simulink model "estimation"  (R2024a)
settings: Solver=VariableStepAuto  StartTime=0.0  StopTime=800  RelTol=1e-3
settings Model: NumberOfSteps=2  Creator=sabri  LastModifiedBy=sabri

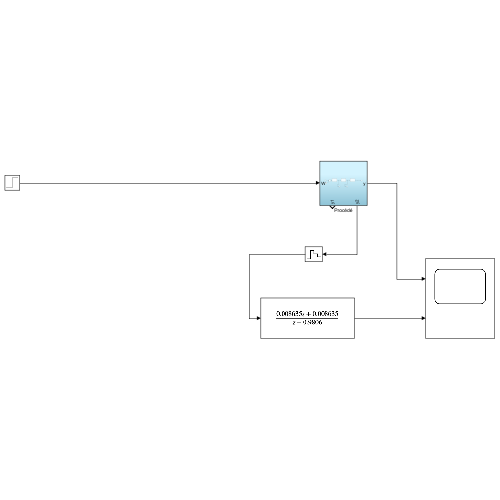
[thumbnail: Simulink's stored preview of the top-level diagram]
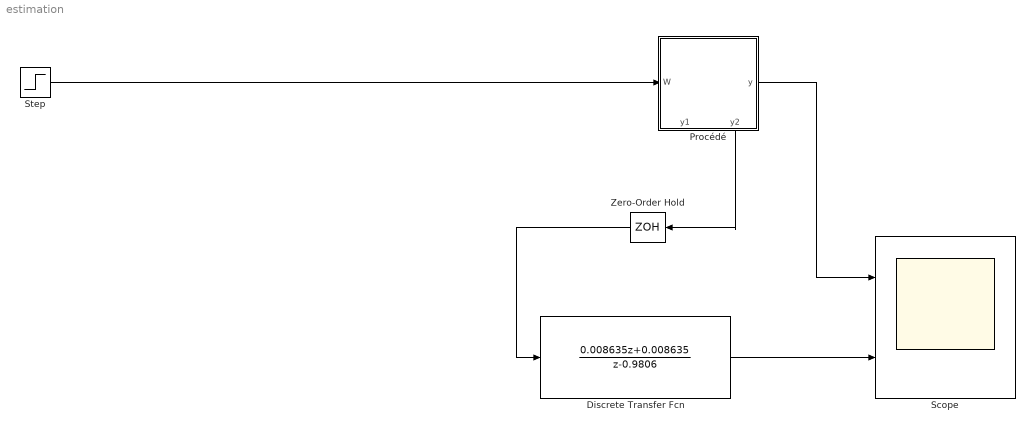
== system estimation ==
  Discrete Transfer Fcn : DiscreteTransferFcn  Numerator=[0.008635 0.008635]  Denominator=[1 -0.9806]
  Procédé : Subsystem
      settings: PortSchema="{\"entries\":[{\"content\":{\"sides\":[{\"content\":{\"connectorIds\":[\"In1\"]},\"type\":\"ConnectorPlacement.EquallySpacedRectSide\",\"uuid\":\"20a23230-a41b-4fdf-8ae4-039aa17abee7\"},{\"content\":{\"connectorIds\":[\"Out1\"],\"side\":\"RIGHT\"},\"type\":\"ConnectorPlacement.EquallySpacedRectSide\",\"uuid\":\"82e4e468-e0ad-4c9f-b6ff-cc9c1ee7ea9d\"},{\"content\":{\"side\":\"TOP\"},\"type\":\"ConnectorPlacement.EquallySpacedRectSide\",\"uuid\":\"049bc4af-9a9a-43aa-9803-dca862d69d2b\"},{\"content\":{\"connectorIds\":[\"Out2\",\"Out3\"],\"side\":\"BOTTOM\"},\"type\":\"ConnectorPlacement.EquallySpacedRectSide\",\"uuid\":\"142d2b37-1c32-477b-9e70-4e4bc8b2913e\"}]},\"type\":\"ConnectorPlacement.EquallySpacedConnector\",\"uuid\":\"a0abf580-2deb-4a1c-9cb8-1272669a26fd\"}],\"packageUris\":[\"http://schema.mathworks.com/mf0/Connector/R2020b\"],\"version\":\"1.0\"}"
  Scope : Scope  NumInputPorts=2
  Step : Step  Time=5  After=10  SampleTime=0
  Zero-Order Hold : ZeroOrderHold  SampleTime=0.5
  wires:
  Discrete Transfer Fcn/1 -> Scope/2
  Procédé/1(y) -> Scope/1
  Procédé/3(y2) -> Zero-Order Hold/1
  Step/1 -> Procédé/1(W)
  Zero-Order Hold/1 -> Discrete Transfer Fcn/1

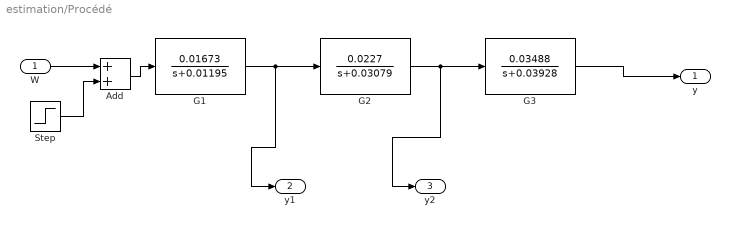
== system estimation/Procédé ==
  W : Inport
  Add : Sum
  G1 : TransferFcn  Numerator=[0.01673]  Denominator=[1 0.01195]
  G2 : TransferFcn  Numerator=[0.0227]  Denominator=[1 0.03079]
  G3 : TransferFcn  Numerator=[0.03488]  Denominator=[1 0.03928]
  Step : Step  Time=60  After=0  SampleTime=0
  y : Outport
  y1 : Outport  Port=2
  y2 : Outport  Port=3
  wires:
  G1/1 -> y1/1, G2/1
  Add/1 -> G1/1
  W/1 -> Add/1
  Step/1 -> Add/2
  G3/1 -> y/1
  G2/1 -> y2/1, G3/1
